simulink model "Estados"  (R2017a)
settings: Solver=VariableStepAuto  StartTime=0.0  StopTime=10.0  RelTol=1e-3
values from neighbouring files (symbols this model uses):
  A = [0 1;-k/m -b/m]    [Estados.m]
  B = [0;1/m]    [Estados.m]
  C = [1 0;0 1]    [Estados.m]
settings Model: Creator=franj  LastModifiedBy=franj

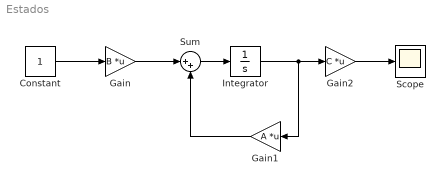
== system Estados ==
  Constant : Constant
  Gain : Gain  Gain=B  Multiplication=Matrix(K*u)
  Gain1 : Gain  Gain=A  Multiplication=Matrix(K*u)
  Gain2 : Gain  Gain=C  Multiplication=Matrix(K*u)
  Integrator : Integrator
  Scope : Scope
  Sum : Sum  Inputs=|++
  wires:
  Gain1/1 -> Sum/2
  Integrator/1 -> Gain2/1, Gain1/1
  Sum/1 -> Integrator/1
  Gain/1 -> Sum/1
  Constant/1 -> Gain/1
  Gain2/1 -> Scope/1
